simulink model "TCMSSystem"  (R2019b)
settings: configuration reference "ConfigSet_TCMSSystem_Reference" (kept outside this file)
model workspace (MAT data in the model file):
  Prm_TCMSSystem : Simulink.Parameter (value not decoded)
  SampleTime = 0.05
symbols that are objects in the model workspace (value not decoded): Prm_TCMSSystem
undefined symbols (not defined in the file): ADDIntervention, AK1Status, AK2Status, AKContactorStatus, AllDoorsClosed, AllLeftDoorsClosed, AllRightDoorsClosed, APS1Fault, APS1Isolated, APS1OutputVoltage, APS1Status, APS2Fault, APS2Isolated, APS2OutputVoltage, APS2Status, APSKAKContactor, ASCOEnd1, ASCOEnd2, ATBMode, ATCBypassMode, ATCStatusNotOK, ATOMode, ATPLowSpeedCutoutStatus, ATPMode, AuxCompressor, BatteryCurrent, BatteryIsolationContactor, BatteryTemperature, BatteryVoltage, BCG1Fault, BCG1Isolated, BCG1IsolationFailed, BCG1OutputCurrent, BCG1Status, BCG2Fault, BCG2Isolated, BCG2OutputCurrent, BCG2Status, BCGOutputVoltage, BECU1AxleLockedWheelSet1, BECU2AxleLockedWheelSet2, BECUFaulty, BECUMajorFault, BECUMinorFault, BECUStatus, BIC1Inside, BIC1Outside, BIC2Inside, BIC2Outside, Bogie, Bogie1WSPStatus, Bogie2WSPStatus, BogieFaulty, BogieIsolationStatus, BogieSupportedMass, BrakeCylinderPressureGauge, BrakeLoopCBTripped, BrakeLoopOpenTL, BrakeTrainLineStatus, BrakingDemand ... (+215)
libraries: TimersLib x257, simulink x137, LatchesLib x42, VectorOperationsLib x15, TestBenchLib x12, MathOperationsLib x2, FiltersLib x1
(part 8 of 16)

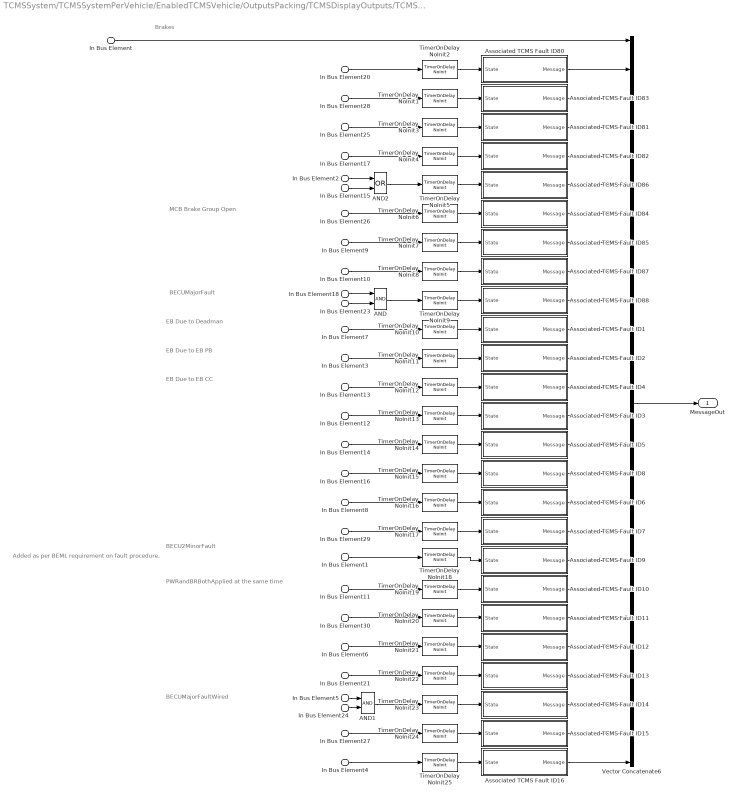
== system TCMSSystem/TCMSSystemPerVehicle/EnabledTCMSVehicle/OutputsPacking/TCMSDisplayOutputs/TCMSMessageEvents/BrakeSystemFaults ==
  note: Added as per BEML requirement on fault procedure.
  note: Brakes
  note: EB Due to Deadman
  note: EB Due to EB PB
  note: EB Due to EB CC
  note: MCB Brake Group Open
  note: PWRandBRBothApplied at the same time
  note: BECUMajorFaultWired
  note: BECU2MinorFault
  note: BECUMajorFault
  In Bus Element : Inport  PortName=MessageIn
  In Bus Element7 : Inport  Port=2  PortName=BusIn  Element=ElectricalSystem.EBDueToDeadman
  In Bus Element3 : Inport  Port=2  PortName=BusIn  Element=ElectricalSystem.EBDueToPushButton
  In Bus Element13 : Inport  Port=2  PortName=BusIn  Element=ElectricalSystem.EBByCC
  In Bus Element9 : Inport  Port=2  PortName=BusIn  Element=PneumaticsSystem.ParkBrakeApplyFailure
  In Bus Element10 : Inport  Port=2  PortName=BusIn  Element=PneumaticsSystem.ParkBrakeReleaseFailure
  In Bus Element25 : Inport  Port=2  PortName=BusIn  Element=PneumaticsSystem.BECU1EmergencyBrakeFailure
  In Bus Element27 : Inport  Port=2  PortName=BusIn  Element=PneumaticsSystem.BECU2EmergencyBrakeFailure
  In Bus Element28 : Inport  Port=2  PortName=BusIn  Element=PneumaticsSystem.BECU1ServiceBrakeFailure
  In Bus Element29 : Inport  Port=2  PortName=BusIn  Element=PneumaticsSystem.BECU1BrakeNotApplied
  In Bus Element30 : Inport  Port=2  PortName=BusIn  Element=PneumaticsSystem.BECU1BrakeNotReleased
  In Bus Element4 : Inport  Port=2  PortName=BusIn  Element=PneumaticsSystem.BECU2CarLoadPressureLow
  In Bus Element8 : Inport  Port=2  PortName=BusIn  Element=PneumaticsSystem.BECU1CarLoadPressureLow
  In Bus Element16 : Inport  Port=2  PortName=BusIn  Element=PneumaticsSystem.BECU1LoadPressureLow
  In Bus Element17 : Inport  Port=2  PortName=BusIn  Element=PneumaticsSystem.AirSuspensionBogie1Deflated
  In Bus Element6 : Inport  Port=2  PortName=BusIn  Element=PneumaticsSystem.BECULowRPressure
  In Bus Element2 : Inport  Port=2  PortName=BusIn  Element=TractionBraking.Bogie1WSPStatus
  In Bus Element15 : Inport  Port=2  PortName=BusIn  Element=TractionBraking.HeavyWheelSlipDetected
  In Bus Element1 : Inport  Port=2  PortName=BusIn  Element=TractionBraking.BECUMinorFault
  In Bus Element11 : Inport  Port=3  PortName=TractionControl  Element=PWRandBRKBothApplied
  In Bus Element5 : Inport  Port=3  PortName=TractionControl  Element=BECUFaulty
  In Bus Element18 : Inport  Port=3  PortName=TractionControl  Element=BECUFaulty
  In Bus Element14 : Inport  Port=3  PortName=TractionControl  Element=SpeedSensorFault
  In Bus Element20 : Inport  Port=3  PortName=TractionControl  Element=BECU1AxleLockedWheelSet1
  In Bus Element21 : Inport  Port=3  PortName=TractionControl  Element=BECU2AxleLockedWheelSet2
  In Bus Element23 : Inport  Port=4  PortName=TCMSFaults  Element=BECUMajorFault
  In Bus Element24 : Inport  Port=4  PortName=TCMSFaults  Element=BECUMajorFaultWired
  In Bus Element12 : Inport  Port=5  PortName=VehicleLevelFaults  Element=BECU1MissingOnSegment
  In Bus Element26 : Inport  Port=6  PortName=ElectricalControl  Element=MCBBrakeGroup
  AND : Logic  AllPortsSameDT=off  OutDataTypeStr=boolean
  AND1 : Logic  AllPortsSameDT=off  OutDataTypeStr=boolean
  AND2 : Logic  Operator=OR  AllPortsSameDT=off  OutDataTypeStr=boolean
  Associated TCMS Fault ID1 : Subsystem  mask{MessageID=091046}
      mask Display:
      | port_label('output', 1, ['ID = ' num2str(MessageID)])
      | port_label('input', 1, 'Status')
  Associated TCMS Fault ID10 : Subsystem  mask{MessageID=091052}
      mask Display:
      | port_label('output', 1, ['ID = ' num2str(MessageID)])
      | port_label('input', 1, 'Status')
  Associated TCMS Fault ID11 : Subsystem  mask{MessageID=091053}
      mask Display:
      | port_label('output', 1, ['ID = ' num2str(MessageID)])
      | port_label('input', 1, 'Status')
  Associated TCMS Fault ID12 : Subsystem  mask{MessageID=091004}
      mask Display:
      | port_label('output', 1, ['ID = ' num2str(MessageID)])
      | port_label('input', 1, 'Status')
  Associated TCMS Fault ID13 : Subsystem  mask{MessageID=092009}
      mask Display:
      | port_label('output', 1, ['ID = ' num2str(MessageID)])
      | port_label('input', 1, 'Status')
  Associated TCMS Fault ID14 : Subsystem  mask{MessageID=091051}
      mask Display:
      | port_label('output', 1, ['ID = ' num2str(MessageID)])
      | port_label('input', 1, 'Status')
  Associated TCMS Fault ID15 : Subsystem  mask{MessageID=091019}
      mask Display:
      | port_label('output', 1, ['ID = ' num2str(MessageID)])
      | port_label('input', 1, 'Status')
  Associated TCMS Fault ID16 : Subsystem  mask{MessageID=091015}
      mask Display:
      | port_label('output', 1, ['ID = ' num2str(MessageID)])
      | port_label('input', 1, 'Status')
  Associated TCMS Fault ID2 : Subsystem  mask{MessageID=091044}
      mask Display:
      | port_label('output', 1, ['ID = ' num2str(MessageID)])
      | port_label('input', 1, 'Status')
  Associated TCMS Fault ID3 : Subsystem  mask{MessageID=091001}
      mask Display:
      | port_label('output', 1, ['ID = ' num2str(MessageID)])
      | port_label('input', 1, 'Status')
  Associated TCMS Fault ID4 : Subsystem  mask{MessageID=090043}
      mask Display:
      | port_label('output', 1, ['ID = ' num2str(MessageID)])
      | port_label('input', 1, 'Status')
  Associated TCMS Fault ID5 : Subsystem  mask{MessageID=091005}
      mask Display:
      | port_label('output', 1, ['ID = ' num2str(MessageID)])
      | port_label('input', 1, 'Status')
  Associated TCMS Fault ID6 : Subsystem  mask{MessageID=091014}
      mask Display:
      | port_label('output', 1, ['ID = ' num2str(MessageID)])
      | port_label('input', 1, 'Status')
  Associated TCMS Fault ID7 : Subsystem  mask{MessageID=091020}
      mask Display:
      | port_label('output', 1, ['ID = ' num2str(MessageID)])
      | port_label('input', 1, 'Status')
  Associated TCMS Fault ID8 : Subsystem  mask{MessageID=091012}
      mask Display:
      | port_label('output', 1, ['ID = ' num2str(MessageID)])
      | port_label('input', 1, 'Status')
  Associated TCMS Fault ID80 : Subsystem  mask{MessageID=091008}
      mask Display:
      | port_label('output', 1, ['ID = ' num2str(MessageID)])
      | port_label('input', 1, 'Status')
  Associated TCMS Fault ID81 : Subsystem  mask{MessageID=091018}
      mask Display:
      | port_label('output', 1, ['ID = ' num2str(MessageID)])
      | port_label('input', 1, 'Status')
  Associated TCMS Fault ID82 : Subsystem  mask{MessageID=091038}
      mask Display:
      | port_label('output', 1, ['ID = ' num2str(MessageID)])
      | port_label('input', 1, 'Status')
  Associated TCMS Fault ID83 : Subsystem  mask{MessageID=091016}
      mask Display:
      | port_label('output', 1, ['ID = ' num2str(MessageID)])
      | port_label('input', 1, 'Status')
  Associated TCMS Fault ID84 : Subsystem  mask{MessageID=091042}
      mask Display:
      | port_label('output', 1, ['ID = ' num2str(MessageID)])
      | port_label('input', 1, 'Status')
  Associated TCMS Fault ID85 : Subsystem  mask{MessageID=091048}
      mask Display:
      | port_label('output', 1, ['ID = ' num2str(MessageID)])
      | port_label('input', 1, 'Status')
  Associated TCMS Fault ID86 : Subsystem  mask{MessageID=091040}
      mask Display:
      | port_label('output', 1, ['ID = ' num2str(MessageID)])
      | port_label('input', 1, 'Status')
  Associated TCMS Fault ID87 : Subsystem  mask{MessageID=091049}
      mask Display:
      | port_label('output', 1, ['ID = ' num2str(MessageID)])
      | port_label('input', 1, 'Status')
  Associated TCMS Fault ID88 : Subsystem  mask{MessageID=091050}
      mask Display:
      | port_label('output', 1, ['ID = ' num2str(MessageID)])
      | port_label('input', 1, 'Status')
  Associated TCMS Fault ID9 : Subsystem  mask{MessageID=091023}
      mask Display:
      | port_label('output', 1, ['ID = ' num2str(MessageID)])
      | port_label('input', 1, 'Status')
  TimerOnDelay NoInit{1..25} (25 alike) : TimersLib/TimerOnDelay NoInit  UpperSaturationLimit=0.5  OutputTime=off  SampleTime=-1
      settings: SourceProductName=Sydac Utilities
  Vector Concatenate6 : Concatenate  NumInputs=26
  MessageOut : Outport
  wires:
  Associated TCMS Fault ID82/1(Message) -> Vector Concatenate6/5
  Associated TCMS Fault ID80/1(Message) -> Vector Concatenate6/2
  Associated TCMS Fault ID85/1(Message) -> Vector Concatenate6/8
  Associated TCMS Fault ID84/1(Message) -> Vector Concatenate6/7
  Associated TCMS Fault ID83/1(Message) -> Vector Concatenate6/3
  Associated TCMS Fault ID86/1(Message) -> Vector Concatenate6/6
  Associated TCMS Fault ID88/1(Message) -> Vector Concatenate6/10
  Associated TCMS Fault ID87/1(Message) -> Vector Concatenate6/9
  Associated TCMS Fault ID81/1(Message) -> Vector Concatenate6/4
  Vector Concatenate6/1 -> MessageOut/1
  In Bus Element/1 -> Vector Concatenate6/1
  In Bus Element20/1 -> TimerOnDelay NoInit2/1
  In Bus Element28/1 -> TimerOnDelay NoInit1/1
  In Bus Element25/1 -> TimerOnDelay NoInit3/1
  AND/1 -> TimerOnDelay NoInit9/1
  In Bus Element17/1 -> TimerOnDelay NoInit4/1
  In Bus Element2/1 -> AND2/1
  In Bus Element26/1 -> TimerOnDelay NoInit6/1
  In Bus Element9/1 -> TimerOnDelay NoInit7/1
  In Bus Element10/1 -> TimerOnDelay NoInit8/1
  In Bus Element7/1 -> TimerOnDelay NoInit10/1
  Associated TCMS Fault ID1/1(Message) -> Vector Concatenate6/11
  Associated TCMS Fault ID2/1(Message) -> Vector Concatenate6/12
  In Bus Element3/1 -> TimerOnDelay NoInit11/1
  In Bus Element13/1 -> TimerOnDelay NoInit12/1
  Associated TCMS Fault ID4/1(Message) -> Vector Concatenate6/13
  In Bus Element29/1 -> TimerOnDelay NoInit17/1
  In Bus Element8/1 -> TimerOnDelay NoInit16/1
  In Bus Element16/1 -> TimerOnDelay NoInit15/1
  In Bus Element14/1 -> TimerOnDelay NoInit14/1
  In Bus Element11/1 -> TimerOnDelay NoInit19/1
  In Bus Element12/1 -> TimerOnDelay NoInit13/1
  Associated TCMS Fault ID3/1(Message) -> Vector Concatenate6/14
  Associated TCMS Fault ID9/1(Message) -> Vector Concatenate6/19
  Associated TCMS Fault ID10/1(Message) -> Vector Concatenate6/20
  Associated TCMS Fault ID8/1(Message) -> Vector Concatenate6/16
  Associated TCMS Fault ID6/1(Message) -> Vector Concatenate6/17
  Associated TCMS Fault ID7/1(Message) -> Vector Concatenate6/18
  Associated TCMS Fault ID5/1(Message) -> Vector Concatenate6/15
  Associated TCMS Fault ID11/1(Message) -> Vector Concatenate6/21
  In Bus Element30/1 -> TimerOnDelay NoInit20/1
  In Bus Element6/1 -> TimerOnDelay NoInit21/1
  In Bus Element21/1 -> TimerOnDelay NoInit22/1
  Associated TCMS Fault ID13/1(Message) -> Vector Concatenate6/23
  Associated TCMS Fault ID12/1(Message) -> Vector Concatenate6/22
  Associated TCMS Fault ID14/1(Message) -> Vector Concatenate6/24
  In Bus Element24/1 -> AND1/2
  In Bus Element23/1 -> AND/2
  AND1/1 -> TimerOnDelay NoInit23/1
  In Bus Element5/1 -> AND1/1
  In Bus Element18/1 -> AND/1
  In Bus Element27/1 -> TimerOnDelay NoInit24/1
  Associated TCMS Fault ID15/1(Message) -> Vector Concatenate6/25
  In Bus Element4/1 -> TimerOnDelay NoInit25/1
  Associated TCMS Fault ID16/1(Message) -> Vector Concatenate6/26
  TimerOnDelay NoInit2/1 -> Associated TCMS Fault ID80/1(State)
  TimerOnDelay NoInit1/1 -> Associated TCMS Fault ID83/1(State)
  TimerOnDelay NoInit3/1 -> Associated TCMS Fault ID81/1(State)
  TimerOnDelay NoInit4/1 -> Associated TCMS Fault ID82/1(State)
  TimerOnDelay NoInit5/1 -> Associated TCMS Fault ID86/1(State)
  TimerOnDelay NoInit6/1 -> Associated TCMS Fault ID84/1(State)
  TimerOnDelay NoInit7/1 -> Associated TCMS Fault ID85/1(State)
  TimerOnDelay NoInit8/1 -> Associated TCMS Fault ID87/1(State)
  TimerOnDelay NoInit9/1 -> Associated TCMS Fault ID88/1(State)
  TimerOnDelay NoInit10/1 -> Associated TCMS Fault ID1/1(State)
  TimerOnDelay NoInit11/1 -> Associated TCMS Fault ID2/1(State)
  TimerOnDelay NoInit12/1 -> Associated TCMS Fault ID4/1(State)
  TimerOnDelay NoInit13/1 -> Associated TCMS Fault ID3/1(State)
  TimerOnDelay NoInit14/1 -> Associated TCMS Fault ID5/1(State)
  TimerOnDelay NoInit15/1 -> Associated TCMS Fault ID8/1(State)
  TimerOnDelay NoInit16/1 -> Associated TCMS Fault ID6/1(State)
  TimerOnDelay NoInit17/1 -> Associated TCMS Fault ID7/1(State)
  TimerOnDelay NoInit18/1 -> Associated TCMS Fault ID9/1(State)
  TimerOnDelay NoInit19/1 -> Associated TCMS Fault ID10/1(State)
  TimerOnDelay NoInit20/1 -> Associated TCMS Fault ID11/1(State)
  TimerOnDelay NoInit21/1 -> Associated TCMS Fault ID12/1(State)
  TimerOnDelay NoInit22/1 -> Associated TCMS Fault ID13/1(State)
  TimerOnDelay NoInit23/1 -> Associated TCMS Fault ID14/1(State)
  TimerOnDelay NoInit24/1 -> Associated TCMS Fault ID15/1(State)
  TimerOnDelay NoInit25/1 -> Associated TCMS Fault ID16/1(State)
  AND2/1 -> TimerOnDelay NoInit5/1
  In Bus Element15/1 -> AND2/2
  In Bus Element1/1 -> TimerOnDelay NoInit18/1

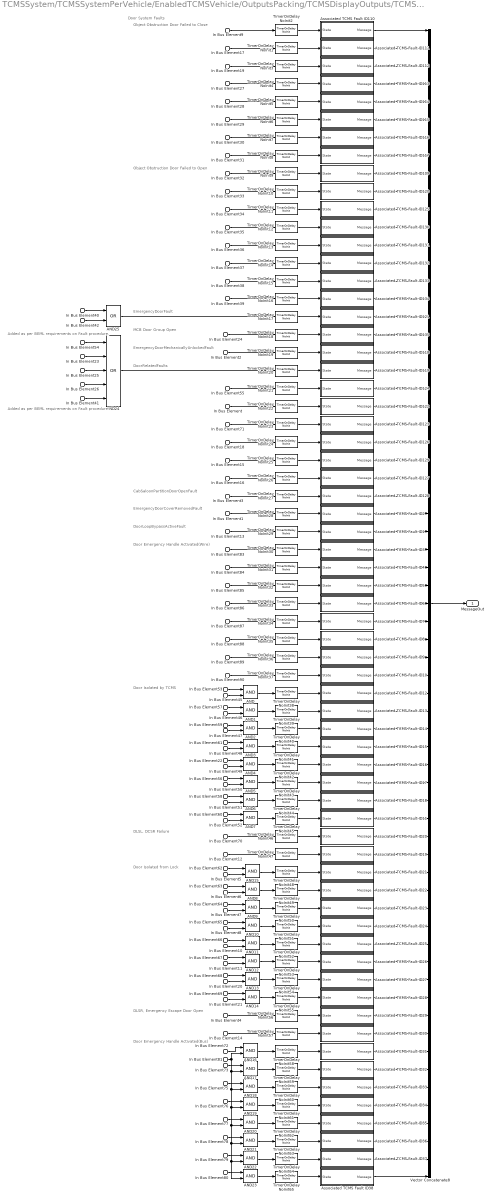
== system TCMSSystem/TCMSSystemPerVehicle/EnabledTCMSVehicle/OutputsPacking/TCMSDisplayOutputs/TCMSMessageEvents/DoorSystemFaults ==
  note: Added as per BEML requirements on Fault procedure.
  note: Object Obstruction Door Failed to Close
  note: Door System Faults
  note: Object Obstruction Door Failed to Open
  note: EmergencyDoorFault
  note: CabSaloonPartitionDoorOpenFault
  note: EmergencyDoorMechanicallyUnlockedFault
  note: EmergencyDoorCoverRemovedFault
  note: DoorLoopBypassActiveFault
  note: Door Emergency Handle Activated(Wire)
  note: Door Isolated by TCMS
  note: MCB Door Group Open
  note: DoorRelatedFaults
  note: Door Isolated from Lock
  note: DLSR, Emergency Escape Door Open
  note: DLSL, DCSR Failure
  note: Door Emergency Handle Activated(Bus)
  note: Added as per BEML requirements on Fault procedure.
  In Bus Element9 : Inport  PortName=BusIn  Element=DoorSystem.Doors.DoorA1CloseObstruction
  In Bus Element17 : Inport  PortName=BusIn  Element=DoorSystem.Doors.DoorA2CloseObstruction
  In Bus Element19 : Inport  PortName=BusIn  Element=DoorSystem.Doors.DoorA3CloseObstruction
  In Bus Element27 : Inport  PortName=BusIn  Element=DoorSystem.Doors.DoorA4CloseObstruction
  In Bus Element28 : Inport  PortName=BusIn  Element=DoorSystem.Doors.DoorB1CloseObstruction
  In Bus Element29 : Inport  PortName=BusIn  Element=DoorSystem.Doors.DoorB2CloseObstruction
  In Bus Element30 : Inport  PortName=BusIn  Element=DoorSystem.Doors.DoorB3CloseObstruction
  In Bus Element31 : Inport  PortName=BusIn  Element=DoorSystem.Doors.DoorB4CloseObstruction
  In Bus Element32 : Inport  PortName=BusIn  Element=DoorSystem.Doors.DoorA1OpenObstruction
  In Bus Element33 : Inport  PortName=BusIn  Element=DoorSystem.Doors.DoorA2OpenObstruction
  In Bus Element34 : Inport  PortName=BusIn  Element=DoorSystem.Doors.DoorA3OpenObstruction
  In Bus Element35 : Inport  PortName=BusIn  Element=DoorSystem.Doors.DoorA4OpenObstruction
  In Bus Element36 : Inport  PortName=BusIn  Element=DoorSystem.Doors.DoorB1OpenObstruction
  In Bus Element37 : Inport  PortName=BusIn  Element=DoorSystem.Doors.DoorB2OpenObstruction
  In Bus Element38 : Inport  PortName=BusIn  Element=DoorSystem.Doors.DoorB3OpenObstruction
  In Bus Element39 : Inport  PortName=BusIn  Element=DoorSystem.Doors.DoorB4OpenObstruction
  In Bus Element72 : Inport  PortName=BusIn  Element=DoorSystem.Doors.DoorA1EmergencyReleased
  In Bus Element73 : Inport  PortName=BusIn  Element=DoorSystem.Doors.DoorA2EmergencyReleased
  In Bus Element75 : Inport  PortName=BusIn  Element=DoorSystem.Doors.DoorA3EmergencyReleased
  In Bus Element76 : Inport  PortName=BusIn  Element=DoorSystem.Doors.DoorA4EmergencyReleased
  In Bus Element77 : Inport  PortName=BusIn  Element=DoorSystem.Doors.DoorB1EmergencyReleased
  In Bus Element78 : Inport  PortName=BusIn  Element=DoorSystem.Doors.DoorB2EmergencyReleased
  In Bus Element79 : Inport  PortName=BusIn  Element=DoorSystem.Doors.DoorB3EmergencyReleased
  In Bus Element80 : Inport  PortName=BusIn  Element=DoorSystem.Doors.DoorB4EmergencyReleased
  In Bus Element45 : Inport  PortName=BusIn  Element=DoorSystem.Doors.DoorA1Isolated
  In Bus Element5 : Inport  PortName=BusIn  Element=DoorSystem.Doors.DoorA1Isolated
  In Bus Element46 : Inport  PortName=BusIn  Element=DoorSystem.Doors.DoorA2Isolated
  In Bus Element6 : Inport  PortName=BusIn  Element=DoorSystem.Doors.DoorA2Isolated
  In Bus Element47 : Inport  PortName=BusIn  Element=DoorSystem.Doors.DoorA3Isolated
  In Bus Element7 : Inport  PortName=BusIn  Element=DoorSystem.Doors.DoorA3Isolated
  In Bus Element48 : Inport  PortName=BusIn  Element=DoorSystem.Doors.DoorA4Isolated
  In Bus Element8 : Inport  PortName=BusIn  Element=DoorSystem.Doors.DoorA4Isolated
  In Bus Element49 : Inport  PortName=BusIn  Element=DoorSystem.Doors.DoorB1Isolated
  In Bus Element10 : Inport  PortName=BusIn  Element=DoorSystem.Doors.DoorB1Isolated
  In Bus Element50 : Inport  PortName=BusIn  Element=DoorSystem.Doors.DoorB2Isolated
  In Bus Element11 : Inport  PortName=BusIn  Element=DoorSystem.Doors.DoorB2Isolated
  In Bus Element51 : Inport  PortName=BusIn  Element=DoorSystem.Doors.DoorB3Isolated
  In Bus Element20 : Inport  PortName=BusIn  Element=DoorSystem.Doors.DoorB3Isolated
  In Bus Element52 : Inport  PortName=BusIn  Element=DoorSystem.Doors.DoorB4Isolated
  In Bus Element21 : Inport  PortName=BusIn  Element=DoorSystem.Doors.DoorB4Isolated
  In Bus Element : Inport  PortName=BusIn  Element=DoorSystem.Doors.DoorA1MotorCircuitFailure
  In Bus Element15 : Inport  PortName=BusIn  Element=DoorSystem.Doors.DoorA1FailedToLock
  In Bus Element16 : Inport  PortName=BusIn  Element=DoorSystem.Doors.DoorA1FailedToUnlock
  In Bus Element18 : Inport  PortName=BusIn  Element=DoorSystem.Doors.DoorA1UnexpectedUnlocking
  In Bus Element54 : Inport  PortName=BusIn  Element=DoorSystem.Doors.DoorA1DoorMajorFault
  In Bus Element55 : Inport  PortName=BusIn  Element=DoorSystem.Doors.DoorA1DCUFailure
  In Bus Element70 : Inport  PortName=BusIn  Element=DoorSystem.Doors.DoorA1DLSLFailure
  In Bus Element25 : Inport  PortName=BusIn  Element=DoorSystem.Doors.DoorA1DLSLFailure
  In Bus Element12 : Inport  PortName=BusIn  Element=DoorSystem.Doors.DoorA1DCSRFailure
  In Bus Element26 : Inport  PortName=BusIn  Element=DoorSystem.Doors.DoorA1DCSRFailure
  In Bus Element71 : Inport  PortName=BusIn  Element=DoorSystem.Doors.DoorA1DCSLFailure
  In Bus Element23 : Inport  PortName=BusIn  Element=DoorSystem.Doors.DoorA1DCSLFailure
  In Bus Element4 : Inport  PortName=BusIn  Element=DoorSystem.Doors.DoorA1DLSRFailure
  In Bus Element41 : Inport  PortName=BusIn  Element=DoorSystem.Doors.DoorA1DLSRFailure
  In Bus Element83 : Inport  PortName=BusIn  Element=DoorSystem.Doors.DoorA1LocalEED
  In Bus Element84 : Inport  PortName=BusIn  Element=DoorSystem.Doors.DoorA2LocalEED
  In Bus Element85 : Inport  PortName=BusIn  Element=DoorSystem.Doors.DoorA3LocalEED
  In Bus Element86 : Inport  PortName=BusIn  Element=DoorSystem.Doors.DoorA4LocalEED
  In Bus Element87 : Inport  PortName=BusIn  Element=DoorSystem.Doors.DoorB1LocalEED
  In Bus Element88 : Inport  PortName=BusIn  Element=DoorSystem.Doors.DoorB2LocalEED
  In Bus Element89 : Inport  PortName=BusIn  Element=DoorSystem.Doors.DoorB3LocalEED
  In Bus Element90 : Inport  PortName=BusIn  Element=DoorSystem.Doors.DoorB4LocalEED
  In Bus Element40 : Inport  PortName=BusIn  Element=DoorSystem.EmerDoorFaultMessage
  In Bus Element3 : Inport  PortName=BusIn  Element=DoorSystem.CabSaloonPartitionDoorOpen
  In Bus Element1 : Inport  PortName=BusIn  Element=DoorSystem.EmergencyDoorCoverRemoved
  In Bus Element13 : Inport  PortName=BusIn  Element=DoorSystem.DoorLoopBypassActive
  In Bus Element2 : Inport  PortName=BusIn  Element=DoorSystem.EmergencyEscapeDoorUnlocked
  In Bus Element62 : Inport  PortName=BusIn  Element=DoorSystem.LeftDoor1Lockout
  In Bus Element63 : Inport  PortName=BusIn  Element=DoorSystem.LeftDoor2Lockout
  In Bus Element64 : Inport  PortName=BusIn  Element=DoorSystem.LeftDoor3Lockout
  In Bus Element65 : Inport  PortName=BusIn  Element=DoorSystem.LeftDoor4Lockout
  In Bus Element66 : Inport  PortName=BusIn  Element=DoorSystem.RightDoor1Lockout
  In Bus Element67 : Inport  PortName=BusIn  Element=DoorSystem.RightDoor2Lockout
  In Bus Element68 : Inport  PortName=BusIn  Element=DoorSystem.RightDoor3Lockout
  In Bus Element69 : Inport  PortName=BusIn  Element=DoorSystem.RightDoor4Lockout
  In Bus Element14 : Inport  PortName=BusIn  Element=DoorSystem.EmergencyEscapeDoorOpen
  In Bus Element42 : Inport  PortName=BusIn  Element=DoorSystem.EmergencyEscapeDoorOpen
  In Bus Element22 : Inport  Port=2  PortName=DoorsControl  Element=DoorRight1Isolation
  In Bus Element53 : Inport  Port=2  PortName=DoorsControl  Element=DoorLeft1Isolation
  In Bus Element56 : Inport  Port=2  PortName=DoorsControl  Element=DoorRight2Isolation
  In Bus Element57 : Inport  Port=2  PortName=DoorsControl  Element=DoorLeft2Isolation
  In Bus Element58 : Inport  Port=2  PortName=DoorsControl  Element=DoorRight3Isolation
  In Bus Element59 : Inport  Port=2  PortName=DoorsControl  Element=DoorLeft3Isolation
  In Bus Element60 : Inport  Port=2  PortName=DoorsControl  Element=DoorRight4Isolation
  In Bus Element61 : Inport  Port=2  PortName=DoorsControl  Element=DoorLeft4Isolation
  In Bus Element81 : Inport  Port=3  PortName=VehicleFaults  Element=DoorEmergencyHandleActivation
  In Bus Element24 : Inport  Port=4  PortName=ElectricalControl  Element=MCBDoorGroup
  AND{,1..23} (24 alike) : Logic  AllPortsSameDT=off  OutDataTypeStr=boolean
  AND24 : Logic  Operator=OR  Inputs=5  AllPortsSameDT=off  OutDataTypeStr=boolean
  AND25 : Logic  Operator=OR  AllPortsSameDT=off  OutDataTypeStr=boolean
  Associated TCMS Fault ID1 : Subsystem  mask{MessageID=101008}
      mask Display:
      | port_label('output', 1, ['ID = ' num2str(MessageID)])
      | port_label('input', 1, 'Status')
  Associated TCMS Fault ID10 : Subsystem  mask{MessageID=101818}
      mask Display:
      | port_label('output', 1, ['ID = ' num2str(MessageID)])
      | port_label('input', 1, 'Status')
  Associated TCMS Fault ID109 : Subsystem  mask{MessageID=101115}
      mask Display:
      | port_label('output', 1, ['ID = ' num2str(MessageID)])
      | port_label('input', 1, 'Status')
  Associated TCMS Fault ID11 : Subsystem  mask{MessageID=101821}
      mask Display:
      | port_label('output', 1, ['ID = ' num2str(MessageID)])
      | port_label('input', 1, 'Status')
  Associated TCMS Fault ID110 : Subsystem  mask{MessageID=101114}
      mask Display:
      | port_label('output', 1, ['ID = ' num2str(MessageID)])
      | port_label('input', 1, 'Status')
  Associated TCMS Fault ID111 : Subsystem  mask{MessageID=101214}
      mask Display:
      | port_label('output', 1, ['ID = ' num2str(MessageID)])
      | port_label('input', 1, 'Status')
  Associated TCMS Fault ID112 : Subsystem  mask{MessageID=101314}
      mask Display:
      | port_label('output', 1, ['ID = ' num2str(MessageID)])
      | port_label('input', 1, 'Status')
  Associated TCMS Fault ID113 : Subsystem  mask{MessageID=101414}
      mask Display:
      | port_label('output', 1, ['ID = ' num2str(MessageID)])
      | port_label('input', 1, 'Status')
  Associated TCMS Fault ID114 : Subsystem  mask{MessageID=101514}
      mask Display:
      | port_label('output', 1, ['ID = ' num2str(MessageID)])
      | port_label('input', 1, 'Status')
  Associated TCMS Fault ID115 : Subsystem  mask{MessageID=101614}
      mask Display:
      | port_label('output', 1, ['ID = ' num2str(MessageID)])
      | port_label('input', 1, 'Status')
  Associated TCMS Fault ID116 : Subsystem  mask{MessageID=101714}
      mask Display:
      | port_label('output', 1, ['ID = ' num2str(MessageID)])
      | port_label('input', 1, 'Status')
  Associated TCMS Fault ID117 : Subsystem  mask{MessageID=101814}
      mask Display:
      | port_label('output', 1, ['ID = ' num2str(MessageID)])
      | port_label('input', 1, 'Status')
  Associated TCMS Fault ID118 : Subsystem  mask{MessageID=101005}
      mask Display:
      | port_label('output', 1, ['ID = ' num2str(MessageID)])
      | port_label('input', 1, 'Status')
  Associated TCMS Fault ID119 : Subsystem  mask{MessageID=101101}
      mask Display:
      | port_label('output', 1, ['ID = ' num2str(MessageID)])
      | port_label('input', 1, 'Status')
  Associated TCMS Fault ID12 : Subsystem  mask{MessageID=101121}
      mask Display:
      | port_label('output', 1, ['ID = ' num2str(MessageID)])
      | port_label('input', 1, 'Status')
  Associated TCMS Fault ID120 : Subsystem  mask{MessageID=101215}
      mask Display:
      | port_label('output', 1, ['ID = ' num2str(MessageID)])
      | port_label('input', 1, 'Status')
  Associated TCMS Fault ID121 : Subsystem  mask{MessageID=120121}
      mask Display:
      | port_label('output', 1, ['ID = ' num2str(MessageID)])
      | port_label('input', 1, 'Status')
  Associated TCMS Fault ID122 : Subsystem  mask{MessageID=101104}
      mask Display:
      | port_label('output', 1, ['ID = ' num2str(MessageID)])
      | port_label('input', 1, 'Status')
  Associated TCMS Fault ID123 : Subsystem  mask{MessageID=101107}
      mask Display:
      | port_label('output', 1, ['ID = ' num2str(MessageID)])
      | port_label('input', 1, 'Status')
  Associated TCMS Fault ID124 : Subsystem  mask{MessageID=101103}
      mask Display:
      | port_label('output', 1, ['ID = ' num2str(MessageID)])
      | port_label('input', 1, 'Status')
  Associated TCMS Fault ID125 : Subsystem  mask{MessageID=101315}
      mask Display:
      | port_label('output', 1, ['ID = ' num2str(MessageID)])
      | port_label('input', 1, 'Status')
  Associated TCMS Fault ID126 : Subsystem  mask{MessageID=101109}
      mask Display:
      | port_label('output', 1, ['ID = ' num2str(MessageID)])
      | port_label('input', 1, 'Status')
  Associated TCMS Fault ID127 : Subsystem  mask{MessageID=101116}
      mask Display:
      | port_label('output', 1, ['ID = ' num2str(MessageID)])
      | port_label('input', 1, 'Status')
  Associated TCMS Fault ID128 : Subsystem  mask{MessageID=101006}
      mask Display:
      | port_label('output', 1, ['ID = ' num2str(MessageID)])
      | port_label('input', 1, 'Status')
  Associated TCMS Fault ID129 : Subsystem  mask{MessageID=101110}
      mask Display:
      | port_label('output', 1, ['ID = ' num2str(MessageID)])
      | port_label('input', 1, 'Status')
  Associated TCMS Fault ID13 : Subsystem  mask{MessageID=101221}
      mask Display:
      | port_label('output', 1, ['ID = ' num2str(MessageID)])
      | port_label('input', 1, 'Status')
  Associated TCMS Fault ID130 : Subsystem  mask{MessageID=101415}
      mask Display:
      | port_label('output', 1, ['ID = ' num2str(MessageID)])
      | port_label('input', 1, 'Status')
  Associated TCMS Fault ID131 : Subsystem  mask{MessageID=101515}
      mask Display:
      | port_label('output', 1, ['ID = ' num2str(MessageID)])
      | port_label('input', 1, 'Status')
  Associated TCMS Fault ID132 : Subsystem  mask{MessageID=101615}
      mask Display:
      | port_label('output', 1, ['ID = ' num2str(MessageID)])
      | port_label('input', 1, 'Status')
  Associated TCMS Fault ID133 : Subsystem  mask{MessageID=101715}
      mask Display:
      | port_label('output', 1, ['ID = ' num2str(MessageID)])
      | port_label('input', 1, 'Status')
  Associated TCMS Fault ID134 : Subsystem  mask{MessageID=101815}
      mask Display:
      | port_label('output', 1, ['ID = ' num2str(MessageID)])
      | port_label('input', 1, 'Status')
  Associated TCMS Fault ID135 : Subsystem  mask{MessageID=101001}
      mask Display:
      | port_label('output', 1, ['ID = ' num2str(MessageID)])
      | port_label('input', 1, 'Status')
  Associated TCMS Fault ID14 : Subsystem  mask{MessageID=101321}
      mask Display:
      | port_label('output', 1, ['ID = ' num2str(MessageID)])
      | port_label('input', 1, 'Status')
  Associated TCMS Fault ID15 : Subsystem  mask{MessageID=101421}
      mask Display:
      | port_label('output', 1, ['ID = ' num2str(MessageID)])
      | port_label('input', 1, 'Status')
  Associated TCMS Fault ID16 : Subsystem  mask{MessageID=101521}
      mask Display:
      | port_label('output', 1, ['ID = ' num2str(MessageID)])
      | port_label('input', 1, 'Status')
  Associated TCMS Fault ID17 : Subsystem  mask{MessageID=101621}
      mask Display:
      | port_label('output', 1, ['ID = ' num2str(MessageID)])
      | port_label('input', 1, 'Status')
  Associated TCMS Fault ID18 : Subsystem  mask{MessageID=101721}
      mask Display:
      | port_label('output', 1, ['ID = ' num2str(MessageID)])
      | port_label('input', 1, 'Status')
  Associated TCMS Fault ID19 : Subsystem  mask{MessageID=101108}
      mask Display:
      | port_label('output', 1, ['ID = ' num2str(MessageID)])
      | port_label('input', 1, 'Status')
  Associated TCMS Fault ID2 : Subsystem  mask{MessageID=101007}
      mask Display:
      | port_label('output', 1, ['ID = ' num2str(MessageID)])
      | port_label('input', 1, 'Status')
  Associated TCMS Fault ID20 : Subsystem  mask{MessageID=101105}
      mask Display:
      | port_label('output', 1, ['ID = ' num2str(MessageID)])
      | port_label('input', 1, 'Status')
  Associated TCMS Fault ID21 : Subsystem  mask{MessageID=101120}
      mask Display:
      | port_label('output', 1, ['ID = ' num2str(MessageID)])
      | port_label('input', 1, 'Status')
  Associated TCMS Fault ID22 : Subsystem  mask{MessageID=101220}
      mask Display:
      | port_label('output', 1, ['ID = ' num2str(MessageID)])
      | port_label('input', 1, 'Status')
  Associated TCMS Fault ID23 : Subsystem  mask{MessageID=101320}
      mask Display:
      | port_label('output', 1, ['ID = ' num2str(MessageID)])
      | port_label('input', 1, 'Status')
  Associated TCMS Fault ID24 : Subsystem  mask{MessageID=101420}
      mask Display:
      | port_label('output', 1, ['ID = ' num2str(MessageID)])
      | port_label('input', 1, 'Status')
  Associated TCMS Fault ID25 : Subsystem  mask{MessageID=101520}
      mask Display:
      | port_label('output', 1, ['ID = ' num2str(MessageID)])
      | port_label('input', 1, 'Status')
  Associated TCMS Fault ID26 : Subsystem  mask{MessageID=101620}
      mask Display:
      | port_label('output', 1, ['ID = ' num2str(MessageID)])
      | port_label('input', 1, 'Status')
  Associated TCMS Fault ID27 : Subsystem  mask{MessageID=101720}
      mask Display:
      | port_label('output', 1, ['ID = ' num2str(MessageID)])
      | port_label('input', 1, 'Status')
  Associated TCMS Fault ID28 : Subsystem  mask{MessageID=101820}
      mask Display:
      | port_label('output', 1, ['ID = ' num2str(MessageID)])
      | port_label('input', 1, 'Status')
  Associated TCMS Fault ID29 : Subsystem  mask{MessageID=101106}
      mask Display:
      | port_label('output', 1, ['ID = ' num2str(MessageID)])
      | port_label('input', 1, 'Status')
  Associated TCMS Fault ID3 : Subsystem  mask{MessageID=101118}
      mask Display:
      | port_label('output', 1, ['ID = ' num2str(MessageID)])
      | port_label('input', 1, 'Status')
  Associated TCMS Fault ID30 : Subsystem  mask{MessageID=101004}
      mask Display:
      | port_label('output', 1, ['ID = ' num2str(MessageID)])
      | port_label('input', 1, 'Status')
  Associated TCMS Fault ID31 : Subsystem  mask{MessageID=101119}
      mask Display:
      | port_label('output', 1, ['ID = ' num2str(MessageID)])
      | port_label('input', 1, 'Status')
  Associated TCMS Fault ID32 : Subsystem  mask{MessageID=101219}
      mask Display:
      | port_label('output', 1, ['ID = ' num2str(MessageID)])
      | port_label('input', 1, 'Status')
  Associated TCMS Fault ID33 : Subsystem  mask{MessageID=101319}
      mask Display:
      | port_label('output', 1, ['ID = ' num2str(MessageID)])
      | port_label('input', 1, 'Status')
  Associated TCMS Fault ID34 : Subsystem  mask{MessageID=101419}
      mask Display:
      | port_label('output', 1, ['ID = ' num2str(MessageID)])
      | port_label('input', 1, 'Status')
  Associated TCMS Fault ID35 : Subsystem  mask{MessageID=101519}
      mask Display:
      | port_label('output', 1, ['ID = ' num2str(MessageID)])
      | port_label('input', 1, 'Status')
  Associated TCMS Fault ID36 : Subsystem  mask{MessageID=101619}
      mask Display:
      | port_label('output', 1, ['ID = ' num2str(MessageID)])
      | port_label('input', 1, 'Status')
  Associated TCMS Fault ID37 : Subsystem  mask{MessageID=101719}
      mask Display:
      | port_label('output', 1, ['ID = ' num2str(MessageID)])
      | port_label('input', 1, 'Status')
  Associated TCMS Fault ID38 : Subsystem  mask{MessageID=101819}
      mask Display:
      | port_label('output', 1, ['ID = ' num2str(MessageID)])
      | port_label('input', 1, 'Status')
  Associated TCMS Fault ID4 : Subsystem  mask{MessageID=101218}
      mask Display:
      | port_label('output', 1, ['ID = ' num2str(MessageID)])
      | port_label('input', 1, 'Status')
  Associated TCMS Fault ID5 : Subsystem  mask{MessageID=101318}
      mask Display:
      | port_label('output', 1, ['ID = ' num2str(MessageID)])
      | port_label('input', 1, 'Status')
  Associated TCMS Fault ID6 : Subsystem  mask{MessageID=101418}
      mask Display:
      | port_label('output', 1, ['ID = ' num2str(MessageID)])
      | port_label('input', 1, 'Status')
  Associated TCMS Fault ID7 : Subsystem  mask{MessageID=101518}
      mask Display:
      | port_label('output', 1, ['ID = ' num2str(MessageID)])
      | port_label('input', 1, 'Status')
  Associated TCMS Fault ID8 : Subsystem  mask{MessageID=101618}
      mask Display:
      | port_label('output', 1, ['ID = ' num2str(MessageID)])
      | port_label('input', 1, 'Status')
  Associated TCMS Fault ID9 : Subsystem  mask{MessageID=101718}
      mask Display:
      | port_label('output', 1, ['ID = ' num2str(MessageID)])
      | port_label('input', 1, 'Status')
  TimerOnDelay NoInit{1..65} (65 alike) : TimersLib/TimerOnDelay NoInit  UpperSaturationLimit=0.5  OutputTime=off  SampleTime=-1
      settings: SourceProductName=Sydac Utilities
  Vector Concatenate8 : Concatenate  NumInputs=65
  MessageOut : Outport
  wires:
  Associated TCMS Fault ID122/1(Message) -> Vector Concatenate8/22
  In Bus Element27/1 -> TimerOnDelay NoInit4/1
  Associated TCMS Fault ID115/1(Message) -> Vector Concatenate8/6
  Associated TCMS Fault ID121/1(Message) -> Vector Concatenate8/17
  Associated TCMS Fault ID118/1(Message) -> Vector Concatenate8/19
  In Bus Element32/1 -> TimerOnDelay NoInit9/1
  AND25/1 -> TimerOnDelay NoInit17/1
  In Bus Element31/1 -> TimerOnDelay NoInit8/1
  Associated TCMS Fault ID134/1(Message) -> Vector Concatenate8/16
  Associated TCMS Fault ID126/1(Message) -> Vector Concatenate8/24
  Associated TCMS Fault ID124/1(Message) -> Vector Concatenate8/21
  Associated TCMS Fault ID127/1(Message) -> Vector Concatenate8/26
  Associated TCMS Fault ID132/1(Message) -> Vector Concatenate8/14
  Associated TCMS Fault ID116/1(Message) -> Vector Concatenate8/7
  Associated TCMS Fault ID114/1(Message) -> Vector Concatenate8/5
  Associated TCMS Fault ID123/1(Message) -> Vector Concatenate8/23
  Associated TCMS Fault ID135/1(Message) -> Vector Concatenate8/18
  In Bus Element30/1 -> TimerOnDelay NoInit7/1
  Associated TCMS Fault ID120/1(Message) -> Vector Concatenate8/10
  Associated TCMS Fault ID133/1(Message) -> Vector Concatenate8/15
  Associated TCMS Fault ID128/1(Message) -> Vector Concatenate8/27
  Associated TCMS Fault ID129/1(Message) -> Vector Concatenate8/25
  Associated TCMS Fault ID110/1(Message) -> Vector Concatenate8/1
  Associated TCMS Fault ID119/1(Message) -> Vector Concatenate8/20
  In Bus Element35/1 -> TimerOnDelay NoInit12/1
  In Bus Element29/1 -> TimerOnDelay NoInit6/1
  Associated TCMS Fault ID112/1(Message) -> Vector Concatenate8/3
  In Bus Element34/1 -> TimerOnDelay NoInit11/1
  Associated TCMS Fault ID125/1(Message) -> Vector Concatenate8/11
  Associated TCMS Fault ID111/1(Message) -> Vector Concatenate8/2
  In Bus Element9/1 -> TimerOnDelay NoInit2/1
  Associated TCMS Fault ID130/1(Message) -> Vector Concatenate8/12
  Associated TCMS Fault ID117/1(Message) -> Vector Concatenate8/8
  Associated TCMS Fault ID109/1(Message) -> Vector Concatenate8/9
  In Bus Element28/1 -> TimerOnDelay NoInit5/1
  In Bus Element39/1 -> TimerOnDelay NoInit16/1
  In Bus Element19/1 -> TimerOnDelay NoInit3/1
  In Bus Element17/1 -> TimerOnDelay NoInit1/1
  Associated TCMS Fault ID131/1(Message) -> Vector Concatenate8/13
  Associated TCMS Fault ID113/1(Message) -> Vector Concatenate8/4
  In Bus Element33/1 -> TimerOnDelay NoInit10/1
  In Bus Element38/1 -> TimerOnDelay NoInit15/1
  In Bus Element36/1 -> TimerOnDelay NoInit13/1
  Vector Concatenate8/1 -> MessageOut/1
  In Bus Element37/1 -> TimerOnDelay NoInit14/1
  In Bus Element24/1 -> TimerOnDelay NoInit18/1
  In Bus Element54/1 -> AND24/1
  In Bus Element55/1 -> TimerOnDelay NoInit21/1
  In Bus Element/1 -> TimerOnDelay NoInit22/1
  In Bus Element71/1 -> TimerOnDelay NoInit23/1
  In Bus Element18/1 -> TimerOnDelay NoInit24/1
  In Bus Element15/1 -> TimerOnDelay NoInit25/1
  In Bus Element16/1 -> TimerOnDelay NoInit26/1
  In Bus Element3/1 -> TimerOnDelay NoInit27/1
  In Bus Element2/1 -> TimerOnDelay NoInit19/1
  In Bus Element1/1 -> TimerOnDelay NoInit28/1
  Associated TCMS Fault ID2/1(Message) -> Vector Concatenate8/28
  Associated TCMS Fault ID1/1(Message) -> Vector Concatenate8/29
  In Bus Element13/1 -> TimerOnDelay NoInit29/1
  Associated TCMS Fault ID10/1(Message) -> Vector Concatenate8/37
  Associated TCMS Fault ID4/1(Message) -> Vector Concatenate8/31
  In Bus Element84/1 -> TimerOnDelay NoInit31/1
  Associated TCMS Fault ID3/1(Message) -> Vector Concatenate8/30
  In Bus Element90/1 -> TimerOnDelay NoInit37/1
  Associated TCMS Fault ID9/1(Message) -> Vector Concatenate8/36
  Associated TCMS Fault ID7/1(Message) -> Vector Concatenate8/34
  Associated TCMS Fault ID5/1(Message) -> Vector Concatenate8/32
  In Bus Element87/1 -> TimerOnDelay NoInit34/1
  In Bus Element88/1 -> TimerOnDelay NoInit35/1
  In Bus Element86/1 -> TimerOnDelay NoInit33/1
  Associated TCMS Fault ID8/1(Message) -> Vector Concatenate8/35
  In Bus Element89/1 -> TimerOnDelay NoInit36/1
  In Bus Element85/1 -> TimerOnDelay NoInit32/1
  Associated TCMS Fault ID6/1(Message) -> Vector Concatenate8/33
  Associated TCMS Fault ID15/1(Message) -> Vector Concatenate8/41
  Associated TCMS Fault ID17/1(Message) -> Vector Concatenate8/43
  AND/1 -> TimerOnDelay NoInit38/1
  Associated TCMS Fault ID14/1(Message) -> Vector Concatenate8/40
  Associated TCMS Fault ID16/1(Message) -> Vector Concatenate8/42
  Associated TCMS Fault ID18/1(Message) -> Vector Concatenate8/44
  Associated TCMS Fault ID12/1(Message) -> Vector Concatenate8/38
  Associated TCMS Fault ID13/1(Message) -> Vector Concatenate8/39
  Associated TCMS Fault ID11/1(Message) -> Vector Concatenate8/45
  Associated TCMS Fault ID20/1(Message) -> Vector Concatenate8/46
  Associated TCMS Fault ID19/1(Message) -> Vector Concatenate8/47
  In Bus Element70/1 -> TimerOnDelay NoInit46/1
  In Bus Element12/1 -> TimerOnDelay NoInit47/1
  Associated TCMS Fault ID21/1(Message) -> Vector Concatenate8/48
  Associated TCMS Fault ID22/1(Message) -> Vector Concatenate8/49
  Associated TCMS Fault ID23/1(Message) -> Vector Concatenate8/50
  Associated TCMS Fault ID24/1(Message) -> Vector Concatenate8/51
  Associated TCMS Fault ID25/1(Message) -> Vector Concatenate8/52
  Associated TCMS Fault ID26/1(Message) -> Vector Concatenate8/53
  Associated TCMS Fault ID27/1(Message) -> Vector Concatenate8/54
  Associated TCMS Fault ID28/1(Message) -> Vector Concatenate8/55
  In Bus Element53/1 -> AND/1
  In Bus Element45/1 -> AND/2
  In Bus Element46/1 -> AND1/2
  In Bus Element57/1 -> AND1/1
  AND1/1 -> TimerOnDelay NoInit39/1
  AND2/1 -> TimerOnDelay NoInit40/1
  In Bus Element59/1 -> AND2/1
  In Bus Element47/1 -> AND2/2
  In Bus Element48/1 -> AND3/2
  In Bus Element61/1 -> AND3/1
  AND3/1 -> TimerOnDelay NoInit41/1
  AND7/1 -> TimerOnDelay NoInit45/1
  In Bus Element60/1 -> AND7/1
  In Bus Element52/1 -> AND7/2
  In Bus Element51/1 -> AND6/2
  In Bus Element58/1 -> AND6/1
  AND6/1 -> TimerOnDelay NoInit44/1
  AND5/1 -> TimerOnDelay NoInit43/1
  In Bus Element56/1 -> AND5/1
  In Bus Element50/1 -> AND5/2
  In Bus Element49/1 -> AND4/2
  In Bus Element22/1 -> AND4/1
  AND4/1 -> TimerOnDelay NoInit42/1
  AND11/1 -> TimerOnDelay NoInit52/1
  In Bus Element66/1 -> AND11/1
  In Bus Element10/1 -> AND11/2
  In Bus Element11/1 -> AND12/2
  In Bus Element67/1 -> AND12/1
  AND12/1 -> TimerOnDelay NoInit53/1
  AND13/1 -> TimerOnDelay NoInit54/1
  In Bus Element68/1 -> AND13/1
  In Bus Element20/1 -> AND13/2
  AND10/1 -> TimerOnDelay NoInit51/1
  In Bus Element65/1 -> AND10/1
  In Bus Element8/1 -> AND10/2
  In Bus Element7/1 -> AND9/2
  In Bus Element64/1 -> AND9/1
  AND9/1 -> TimerOnDelay NoInit50/1
  AND8/1 -> TimerOnDelay NoInit49/1
  In Bus Element63/1 -> AND8/1
  In Bus Element6/1 -> AND8/2
  In Bus Element21/1 -> AND14/2
  In Bus Element69/1 -> AND14/1
  AND14/1 -> TimerOnDelay NoInit55/1
  In Bus Element5/1 -> AND15/2
  In Bus Element62/1 -> AND15/1
  AND15/1 -> TimerOnDelay NoInit48/1
  Associated TCMS Fault ID29/1(Message) -> Vector Concatenate8/56
  In Bus Element4/1 -> TimerOnDelay NoInit56/1
  Associated TCMS Fault ID30/1(Message) -> Vector Concatenate8/57
  In Bus Element14/1 -> TimerOnDelay NoInit57/1
  In Bus Element75/1 -> AND18/1
  In Bus Element79/1 -> AND22/1
  In Bus Element76/1 -> AND19/1
  In Bus Element72/1 -> AND16/1
  In Bus Element78/1 -> AND21/1
  In Bus Element77/1 -> AND20/1
  In Bus Element80/1 -> AND23/1
  In Bus Element73/1 -> AND17/1
  Associated TCMS Fault ID31/1(Message) -> Vector Concatenate8/58
  Associated TCMS Fault ID32/1(Message) -> Vector Concatenate8/59
  Associated TCMS Fault ID33/1(Message) -> Vector Concatenate8/60
  Associated TCMS Fault ID34/1(Message) -> Vector Concatenate8/61
  Associated TCMS Fault ID35/1(Message) -> Vector Concatenate8/62
  Associated TCMS Fault ID36/1(Message) -> Vector Concatenate8/63
  Associated TCMS Fault ID37/1(Message) -> Vector Concatenate8/64
  Associated TCMS Fault ID38/1(Message) -> Vector Concatenate8/65
  AND16/1 -> TimerOnDelay NoInit58/1
  AND17/1 -> TimerOnDelay NoInit59/1
  AND18/1 -> TimerOnDelay NoInit60/1
  AND19/1 -> TimerOnDelay NoInit61/1
  AND20/1 -> TimerOnDelay NoInit62/1
  AND21/1 -> TimerOnDelay NoInit63/1
  AND22/1 -> TimerOnDelay NoInit64/1
  AND23/1 -> TimerOnDelay NoInit65/1
  In Bus Element81/1 -> AND19/2, AND20/2, AND21/2, AND22/2, AND23/2, AND18/2, AND17/2, AND16/2
  In Bus Element83/1 -> TimerOnDelay NoInit30/1
  TimerOnDelay NoInit2/1 -> Associated TCMS Fault ID110/1(State)
  TimerOnDelay NoInit1/1 -> Associated TCMS Fault ID111/1(State)
  TimerOnDelay NoInit3/1 -> Associated TCMS Fault ID112/1(State)
  TimerOnDelay NoInit4/1 -> Associated TCMS Fault ID113/1(State)
  TimerOnDelay NoInit5/1 -> Associated TCMS Fault ID114/1(State)
  TimerOnDelay NoInit6/1 -> Associated TCMS Fault ID115/1(State)
  TimerOnDelay NoInit7/1 -> Associated TCMS Fault ID116/1(State)
  TimerOnDelay NoInit8/1 -> Associated TCMS Fault ID117/1(State)
  TimerOnDelay NoInit9/1 -> Associated TCMS Fault ID109/1(State)
  TimerOnDelay NoInit10/1 -> Associated TCMS Fault ID120/1(State)
  TimerOnDelay NoInit11/1 -> Associated TCMS Fault ID125/1(State)
  TimerOnDelay NoInit12/1 -> Associated TCMS Fault ID130/1(State)
  TimerOnDelay NoInit13/1 -> Associated TCMS Fault ID131/1(State)
  TimerOnDelay NoInit14/1 -> Associated TCMS Fault ID132/1(State)
  TimerOnDelay NoInit15/1 -> Associated TCMS Fault ID133/1(State)
  TimerOnDelay NoInit16/1 -> Associated TCMS Fault ID134/1(State)
  TimerOnDelay NoInit17/1 -> Associated TCMS Fault ID121/1(State)
  TimerOnDelay NoInit18/1 -> Associated TCMS Fault ID135/1(State)
  TimerOnDelay NoInit19/1 -> Associated TCMS Fault ID118/1(State)
  TimerOnDelay NoInit20/1 -> Associated TCMS Fault ID119/1(State)
  TimerOnDelay NoInit21/1 -> Associated TCMS Fault ID124/1(State)
  TimerOnDelay NoInit22/1 -> Associated TCMS Fault ID122/1(State)
  TimerOnDelay NoInit23/1 -> Associated TCMS Fault ID123/1(State)
  TimerOnDelay NoInit24/1 -> Associated TCMS Fault ID126/1(State)
  TimerOnDelay NoInit25/1 -> Associated TCMS Fault ID129/1(State)
  TimerOnDelay NoInit26/1 -> Associated TCMS Fault ID127/1(State)
  TimerOnDelay NoInit27/1 -> Associated TCMS Fault ID128/1(State)
  TimerOnDelay NoInit28/1 -> Associated TCMS Fault ID2/1(State)
  TimerOnDelay NoInit29/1 -> Associated TCMS Fault ID1/1(State)
  TimerOnDelay NoInit30/1 -> Associated TCMS Fault ID3/1(State)
  TimerOnDelay NoInit31/1 -> Associated TCMS Fault ID4/1(State)
  TimerOnDelay NoInit32/1 -> Associated TCMS Fault ID5/1(State)
  TimerOnDelay NoInit33/1 -> Associated TCMS Fault ID6/1(State)
  TimerOnDelay NoInit34/1 -> Associated TCMS Fault ID7/1(State)
  TimerOnDelay NoInit35/1 -> Associated TCMS Fault ID8/1(State)
  TimerOnDelay NoInit36/1 -> Associated TCMS Fault ID9/1(State)
  TimerOnDelay NoInit37/1 -> Associated TCMS Fault ID10/1(State)
  TimerOnDelay NoInit38/1 -> Associated TCMS Fault ID12/1(State)
  TimerOnDelay NoInit39/1 -> Associated TCMS Fault ID13/1(State)
  TimerOnDelay NoInit40/1 -> Associated TCMS Fault ID14/1(State)
  TimerOnDelay NoInit41/1 -> Associated TCMS Fault ID15/1(State)
  TimerOnDelay NoInit42/1 -> Associated TCMS Fault ID16/1(State)
  TimerOnDelay NoInit43/1 -> Associated TCMS Fault ID17/1(State)
  TimerOnDelay NoInit44/1 -> Associated TCMS Fault ID18/1(State)
  TimerOnDelay NoInit45/1 -> Associated TCMS Fault ID11/1(State)
  TimerOnDelay NoInit46/1 -> Associated TCMS Fault ID20/1(State)
  TimerOnDelay NoInit47/1 -> Associated TCMS Fault ID19/1(State)
  TimerOnDelay NoInit48/1 -> Associated TCMS Fault ID21/1(State)
  TimerOnDelay NoInit49/1 -> Associated TCMS Fault ID22/1(State)
  TimerOnDelay NoInit50/1 -> Associated TCMS Fault ID23/1(State)
  TimerOnDelay NoInit51/1 -> Associated TCMS Fault ID24/1(State)
  TimerOnDelay NoInit52/1 -> Associated TCMS Fault ID25/1(State)
  TimerOnDelay NoInit53/1 -> Associated TCMS Fault ID26/1(State)
  TimerOnDelay NoInit54/1 -> Associated TCMS Fault ID27/1(State)
  TimerOnDelay NoInit55/1 -> Associated TCMS Fault ID28/1(State)
  TimerOnDelay NoInit56/1 -> Associated TCMS Fault ID29/1(State)
  TimerOnDelay NoInit57/1 -> Associated TCMS Fault ID30/1(State)
  TimerOnDelay NoInit58/1 -> Associated TCMS Fault ID31/1(State)
  TimerOnDelay NoInit59/1 -> Associated TCMS Fault ID32/1(State)
  TimerOnDelay NoInit60/1 -> Associated TCMS Fault ID33/1(State)
  TimerOnDelay NoInit61/1 -> Associated TCMS Fault ID34/1(State)
  TimerOnDelay NoInit62/1 -> Associated TCMS Fault ID35/1(State)
  TimerOnDelay NoInit63/1 -> Associated TCMS Fault ID36/1(State)
  TimerOnDelay NoInit64/1 -> Associated TCMS Fault ID37/1(State)
  TimerOnDelay NoInit65/1 -> Associated TCMS Fault ID38/1(State)
  AND24/1 -> TimerOnDelay NoInit20/1
  In Bus Element23/1 -> AND24/2
  In Bus Element25/1 -> AND24/3
  In Bus Element26/1 -> AND24/4
  In Bus Element41/1 -> AND24/5
  In Bus Element40/1 -> AND25/1
  In Bus Element42/1 -> AND25/2
